simulink model "multi_adder"  (R2024b)
settings: Solver=VariableStepAuto  StartTime=0.0  StopTime=1001  RelTol=1e-3
settings Model: Creator=samue  LastModifiedBy=samue
settings OptimizationCC: BlockReduction=off  ConditionallyExecuteInputs=off  DefaultParameterBehavior=Inlined
settings DebuggingCC: AlgebraicLoopMsg=error
settings HardwareCC: ProdBitPerPointer=32  ProdBitPerSizeT=32  ProdBitPerPtrDiffT=32  ProdLargestAtomicFloat=None  ProdIntDivRoundTo=Undefined  ProdEndianess=Unspecified  ProdWordSize=32  ProdHWDeviceType=ASIC/FPGA->ASIC/FPGA  TargetBitPerPointer=64  TargetBitPerSizeT=64  TargetBitPerPtrDiffT=64  TargetLongLongMode=on  TargetIntDivRoundTo=Zero  TargetEndianess=LittleEndian  TargetWordSize=64  TargetHWDeviceType=Custom Processor->MATLAB Host Computer  ProdEqTarget=off

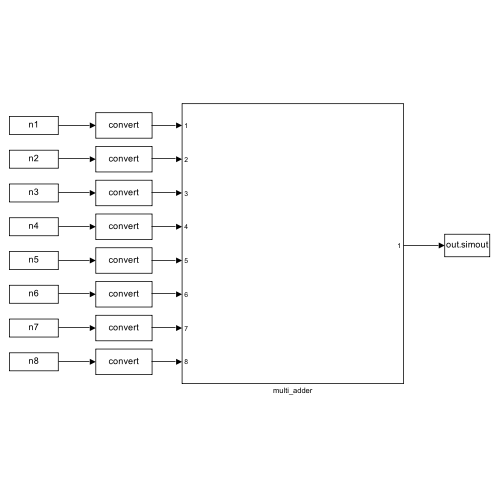
[thumbnail: Simulink's stored preview of the top-level diagram]
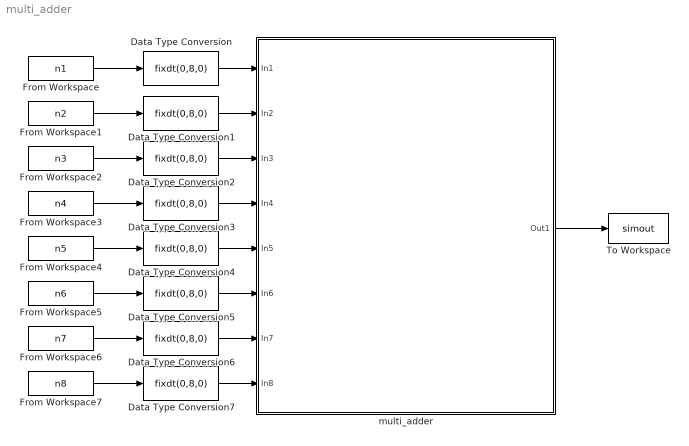
== system multi_adder ==
  Data Type Conversion{,1..4,6..7} (7 alike) : DataTypeConversion  OutDataTypeStr=fixdt(0,8,0)  SaturateOnIntegerOverflow=off  RndMeth=Floor
  Data Type Conversion5 : DataTypeConversion  OutMin=0  OutMax=255  OutDataTypeStr=fixdt(0,8,0)  SaturateOnIntegerOverflow=off  RndMeth=Floor
  From Workspace : FromWorkspace  VariableName=n1  SampleTime=1  Interpolate=off  OutputAfterFinalValue=Holding final value
  From Workspace1 : FromWorkspace  VariableName=n2  SampleTime=1  Interpolate=off  OutputAfterFinalValue=Holding final value
  From Workspace2 : FromWorkspace  VariableName=n3  SampleTime=1  Interpolate=off  OutputAfterFinalValue=Holding final value
  From Workspace3 : FromWorkspace  VariableName=n4  SampleTime=1  Interpolate=off  OutputAfterFinalValue=Holding final value
  From Workspace4 : FromWorkspace  VariableName=n5  SampleTime=1  Interpolate=off  OutputAfterFinalValue=Holding final value
  From Workspace5 : FromWorkspace  VariableName=n6  SampleTime=1  Interpolate=off  OutputAfterFinalValue=Holding final value
  From Workspace6 : FromWorkspace  VariableName=n7  SampleTime=1  Interpolate=off  OutputAfterFinalValue=Holding final value
  From Workspace7 : FromWorkspace  VariableName=n8  SampleTime=1  Interpolate=off  OutputAfterFinalValue=Holding final value
  To Workspace : ToWorkspace  VariableName=simout  SaveFormat=Timeseries  SampleTime=-1
  multi_adder : Subsystem
  wires:
  From Workspace2/1 -> Data Type Conversion2/1
  From Workspace/1 -> Data Type Conversion/1
  From Workspace7/1 -> Data Type Conversion7/1
  From Workspace1/1 -> Data Type Conversion1/1
  From Workspace3/1 -> Data Type Conversion3/1
  From Workspace4/1 -> Data Type Conversion4/1
  From Workspace5/1 -> Data Type Conversion5/1
  From Workspace6/1 -> Data Type Conversion6/1
  multi_adder/1(Out1) -> To Workspace/1
  Data Type Conversion/1 -> multi_adder/1(In1)
  Data Type Conversion1/1 -> multi_adder/2(In2)
  Data Type Conversion2/1 -> multi_adder/3(In3)
  Data Type Conversion3/1 -> multi_adder/4(In4)
  Data Type Conversion4/1 -> multi_adder/5(In5)
  Data Type Conversion5/1 -> multi_adder/6(In6)
  Data Type Conversion6/1 -> multi_adder/7(In7)
  Data Type Conversion7/1 -> multi_adder/8(In8)

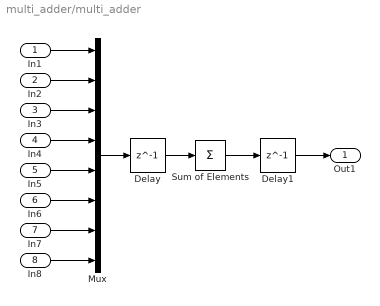
== system multi_adder/multi_adder ==
  In1 : Inport
  In2 : Inport  Port=2
  In3 : Inport  Port=3
  In4 : Inport  Port=4
  In5 : Inport  Port=5
  In6 : Inport  Port=6
  In7 : Inport  Port=7
  In8 : Inport  Port=8
  Delay : Delay  DelayLength=1  InitialCondition=0
  Delay1 : Delay  DelayLength=1  InitialCondition=0
  Mux : Mux  Inputs=8
  Sum of Elements : Sum  Inputs=+  OutDataTypeStr=fixdt(0,11,0)  SaturateOnIntegerOverflow=on
  Out1 : Outport
  wires:
  Sum of Elements/1 -> Delay1/1
  Mux/1 -> Delay/1
  In2/1 -> Mux/2
  In3/1 -> Mux/3
  Delay/1 -> Sum of Elements/1
  In6/1 -> Mux/6
  In8/1 -> Mux/8
  Delay1/1 -> Out1/1
  In5/1 -> Mux/5
  In1/1 -> Mux/1
  In4/1 -> Mux/4
  In7/1 -> Mux/7
